simulink model "five"  (R2020b)
settings: Solver=VariableStepAuto  StartTime=0.0  StopTime=10.0  RelTol=1e-3
model workspace (MAT data in the model file):
  C = Simulink.Parameter
  C.Value = 10
  C.DataType = 'auto'
  C.Dimensions = [1 1]
  R = Simulink.Parameter
  R.Value = 10
  R.DataType = 'auto'
  R.Dimensions = [1 1]
settings Model: Creator=priyaD  LastModifiedBy=priyaD

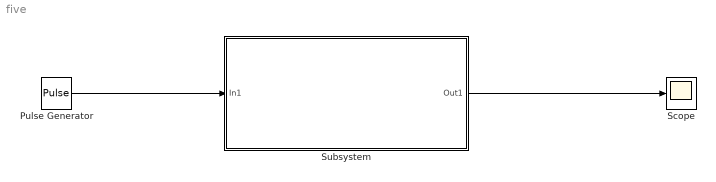
== system five ==
  Pulse Generator : DiscretePulseGenerator  PulseType=Time based  Period=5  PulseWidth=10
  Scope : Scope
  Subsystem : Subsystem
      mask Display: image('C:\Users\priyaD\Desktop\rc.png'); % Use "Edit Image" on toolstrip to change.
  wires:
  Pulse Generator/1 -> Subsystem/1(In1)
  Subsystem/1(Out1) -> Scope/1

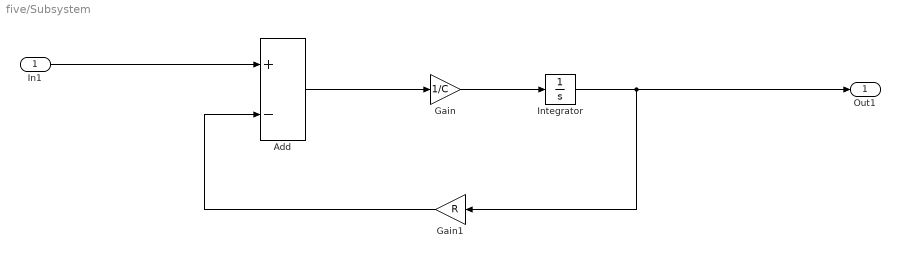
== system five/Subsystem ==
  In1 : Inport
  Add : Sum  Inputs=+-
  Gain : Gain  Gain=1/C
  Gain1 : Gain  Gain=R
  Integrator : Integrator  InitialCondition=0.75
  Out1 : Outport
  wires:
  Add/1 -> Gain/1
  In1/1 -> Add/1
  Integrator/1 -> Out1/1, Gain1/1
  Gain1/1 -> Add/2
  Gain/1 -> Integrator/1
